simulink model "cartpoleSim"  (R2017b)
settings: Solver=VariableStepAuto  StartTime=0.0  StopTime=10.0  RelTol=1e-3
libraries: mpclib x1
settings Model: Creator=janbr  LastModifiedBy=janbr

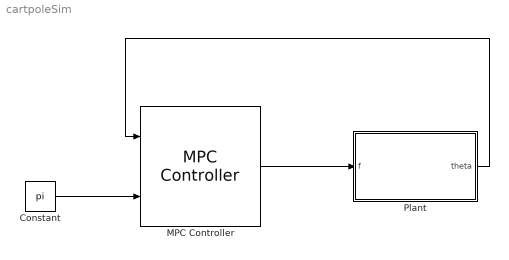
== system cartpoleSim ==
  Constant : Constant  Value=pi
  MPC Controller : mpclib/MPC Controller  SCDEnableBlockLinearizationSpecification=on  mpcobj=mpc1  is_multiple=0  enable_value=0  return_u0=off  ref_from_ws=off  ref_signal_name=[]  ref_preview=off  md_from_ws=off  md_signal_name=[]  md_preview=off  from_project=off  project_file=MPCtask.mat  md_inport=off  mv_inport=off  cost_outport=off  return_sequence=off  return_qpstatus=off  return_state=off  state_inport=off  lims_inport=off  cc_inport=off  ywt_inport=off  is_designfromscratch=0  uwt_inport=off  duwt_inport=off  rhoeps_inport=off  uref_inport=off  n_ts=0.001  n_p=10  n_mv=1  n_md=0  n_ud=0  n_mo=1  n_uo=0  BlockDataType=double  SampleTimeInherited=off  switch_inport=off
  Plant : Subsystem
  wires:
  MPC Controller/1 -> Plant/1(f)
  Constant/1 -> MPC Controller/2
  Plant/1(theta) -> MPC Controller/1

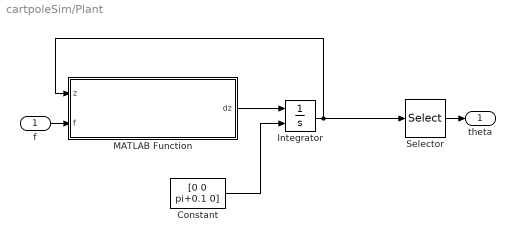
== system cartpoleSim/Plant ==
  f : Inport
  Constant : Constant  Value=[0 0 pi+0.1 0]
  Integrator : Integrator  InitialConditionSource=external
  MATLAB Function : MATLAB Function  TreatAsAtomicUnit=on
  Selector : Selector  InputPortWidth=4  IndexOptions=Index vector (dialog)  Indices=3  OutputSizes=1
  theta : Outport
  wires:
  Integrator/1 -> MATLAB Function/1(z), Selector/1
  f/1 -> MATLAB Function/2(f)
  Selector/1 -> theta/1
  MATLAB Function/1(dz) -> Integrator/1
  Constant/1 -> Integrator/2

== matlab function cartpoleSim/Plant/MATLAB Function ==
  data: z input; dz output; f input
%% dynamics_cp.m
% *Summary:* Implements ths ODE for simulating the cart-pole dynamics.
%
%    function dz = dynamics_cp(t, z, f)
%
%
% *Input arguments:*
%
%   z     state                                                    [4 x 1]
%   f     current force f
%
% *Output arguments:*
%
%   dz    state derivative wrt time
%
%
% Note: It is assumed that the state variables are of the following order:
%       x:        [m]     position of cart
%       dx:       [m/s]   velocity of cart
%       theta:    [rad]   angle
%       dtheta:   [rad/s] angular velocity
%
%
% A detailed derivation of the dynamics can be found in:
%
% M.P. Deisenroth:
% Efficient Reinforcement Learning Using Gaussian Processes, Appendix C,
% KIT Scientific Publishing, 2010.
%
% Copyright (C) 2008-2013 by
% Marc Deisenroth, Andrew McHutchon, Joe Hall, and Carl Edward Rasmussen.
%
% Modified by Matteo Saveriano: 2018-10-17

function dz = dynamics_cart_pole(z,f)
% Parameters
l = 0.5;  % [m]      length of pendulum
m = 0.2;  % [kg]     mass of pendulum
M = 1;  % [kg]     mass of cart
c = 0.2;  % [N/m/s]  coefficient of friction between cart and ground
g = 9.82; % [m/s^2]  acceleration of gravity

dz = zeros(4,1);

% Cart state [x, xd]
dz(1) = z(2);
dz(2) = ( 2*m*l*z(4)^2*sin(z(3)) + 3*m*g*sin(z(3))*cos(z(3)) ...
      + 4*f - 4*c*z(2) )/( 4*(M+m)-3*m*cos(z(3))^2 );
  
% Pole state [theta, dtheta]
dz(3) = z(4);
dz(4) = (-3*m*l*z(4)^2*sin(z(3))*cos(z(3)) - 6*(M+m)*g*sin(z(3)) ...
      - 6*(f-c*z(2))*cos(z(3)) )/( 4*l*(m+M)-3*m*l*cos(z(3))^2 );

% Total Mechanical Energy
%  E = (M+m)*z(2)^2/2 + 1/6*m*l^2*z(3)^2 + m*l*(z(2)*z(3)-g)*cos(z(4))/2;
